simulink model "towing_project"  (Simulink 10.1)
settings: Solver=ode4  StartTime=0.0  StopTime=5000  FixedStep=1  RelTol=1e-3  EnableMultiTasking=on
PreLoadFcn:
  | load('Initialization_data.mat');
values from neighbouring files (symbols this model uses):
  D1 = [MM(1,1)/100, 0, 0; 0, MM(2,2)/40, 0; 0, 0, MM(3,3)/20]    [initail_data.m]
  M1 = diag([6.25e5, 6.25e5, 6.25e5*7.5^2])    [initail_data.m]    (also in msfunMotion_Display.m = makehgtform('translate',[block.Dwork(7).Data(1) block.Dwork()
  Ma1 = [7.58e4, 0, 0; 0, 3.69e5 -1.4e5; 0, -1.4e5, 8.77e6]    [initail_data.m]
  p00 = [0, 0, 0]'    [initail_data.m]
  p10 = [394, 237, 31]'    [initail_data.m]
  p20 = [394, -237, -31]'    [initail_data.m]
  p30 = [-394, -237, -149]'    [initail_data.m]
  p40 = [-394, 237, 149]'    [initail_data.m]
undefined symbols (not defined in the file or in its folder): D, M, Ma, magnitude
libraries: simulink x10, simulink_extras x4
(part 1 of 2)
settings Model: Creator=Lither  LastModifiedBy=Administrator
settings DataIOCC: LimitDataPoints=on
settings OptimizationCC: ExpressionDepthLimit=2147483647
settings DebuggingCC: FcnCallInpInsideContextMsg=warning  StateNameClashWarn=warning
settings ConfigComp: CovSFcnEnable=off

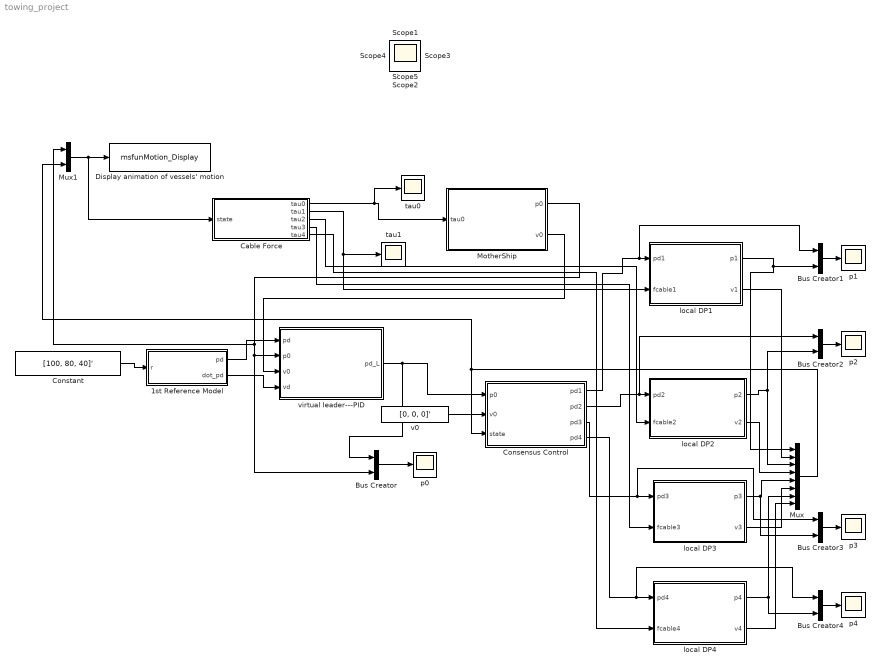
== system towing_project ==
  1st Reference Model : Subsystem  mask{T=200}
      mask prompts: T "Time constant of reference model"
  Bus Creator{,1..4} (5 alike) : BusCreator  Inputs=2
  Cable Force : MATLAB Function  TreatAsAtomicUnit=on
  Consensus Control : MATLAB Function  TreatAsAtomicUnit=on
  Constant : Constant  Value=[100, 80, 40]'
  Display animation of vessels' motion : M-S-Function  FunctionName=msfunMotion_Display  Parameters=p00, p10, p20, p30, p40
  MotherShip : Subsystem  mask{wv=on}
      mask prompts: wv "Display animation of the vessel's motion"
  Mux : Mux  Inputs=8
  Mux1 : Mux  Inputs=2
  local DP1 : Subsystem
  local DP2 : Subsystem
  local DP3 : Subsystem
  local DP4 : Subsystem
  p{0..4} (5 alike) : Scope
  tau0 : Scope
  tau1 : Scope
  v0 : Constant  Value=[0, 0, 0]'
  virtual leader---PID : Subsystem  mask{Kp_L=diag([0.8, 1, 0.8])*0.05, Kd_L=diag([1, 1, 1])*0.03, Ki_L=diag([1, 1, 1])*0.001}
      mask prompts: Kp_L "比例增益：Kp_L"; Kd_L "微分增益：Kd_L"; Ki_L "积分增益：Ki_L"
  Scope{,1..5} (6 alike) : Scope
  wires:
  Consensus Control/1(pd1) -> Bus Creator1/1, local DP1/1(pd1)
  local DP1/1(p1) -> Bus Creator1/2, Mux/1
  local DP1/2(v1) -> Mux/2
  local DP2/1(p2) -> Mux/3, Bus Creator2/2
  local DP2/2(v2) -> Mux/4
  Mux/1 -> Consensus Control/3(state), Mux1/2
  Consensus Control/2(pd2) -> Bus Creator2/1, local DP2/1(pd2)
  Mux1/1 -> Cable Force/1(state), Display animation of vessels' motion/1
  Constant/1 -> 1st Reference Model/1(r)
  local DP3/1(p3) -> Bus Creator3/2, Mux/5
  local DP3/2(v3) -> Mux/6
  local DP4/1(p4) -> Bus Creator4/2, Mux/7
  local DP4/2(v4) -> Mux/8
  Consensus Control/3(pd3) -> Bus Creator3/1, local DP3/1(pd3)
  Consensus Control/4(pd4) -> Bus Creator4/1, local DP4/1(pd4)
  1st Reference Model/1(pd) -> virtual leader---PID/1(pd)
  1st Reference Model/2(dot_pd) -> virtual leader---PID/4(vd)
  virtual leader---PID/1(pd_L) -> Bus Creator/1, Consensus Control/1(p0)
  v0/1 -> Consensus Control/2(v0)
  MotherShip/1(p0) -> Bus Creator/2, virtual leader---PID/2(p0), Mux1/1
  MotherShip/2(v0) -> virtual leader---PID/3(v0)
  Cable Force/1(tau0) -> tau0/1, MotherShip/1(tau0)
  Bus Creator/1 -> p0/1
  Cable Force/2(tau1) -> tau1/1, local DP1/2(fcable1)
  Cable Force/3(tau2) -> local DP2/2(fcable2)
  Cable Force/4(tau3) -> local DP3/2(fcable3)
  Cable Force/5(tau4) -> local DP4/2(fcable4)
  Bus Creator1/1 -> p1/1
  Bus Creator2/1 -> p2/1
  Bus Creator3/1 -> p3/1
  Bus Creator4/1 -> p4/1

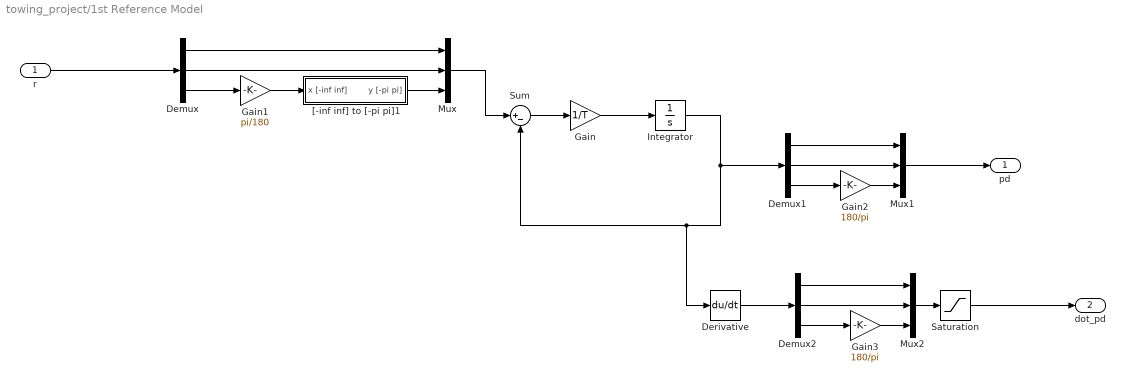
== system towing_project/1st Reference Model ==
  r : Inport
  Demux : Demux  Outputs=3
  Demux1 : Demux  Outputs=3
  Demux2 : Demux  Outputs=3
  Derivative : Derivative
  Gain : Gain  Gain=1/T
  Gain1 : Gain  Gain=pi/180
  Gain2 : Gain  Gain=180/pi
  Gain3 : Gain  Gain=180/pi
  Integrator : Integrator  InitialCondition=p00
  Mux : Mux  Inputs=3
  Mux1 : Mux  Inputs=3
  Mux2 : Mux  Inputs=3
  Saturation : Saturate  UpperLimit=10  LowerLimit=-10
  Sum : Sum  Inputs=|+-
  "[-inf inf] to [-pi pi]1" : Subsystem
  pd : Outport
  dot_pd : Outport  Port=2
  wires:
  Integrator/1 -> Derivative/1, Sum/2, Demux1/1
  Sum/1 -> Gain/1
  Gain/1 -> Integrator/1
  Saturation/1 -> dot_pd/1
  r/1 -> Demux/1
  Demux/3 -> Gain1/1
  Demux/2 -> Mux/2
  Demux/1 -> Mux/1
  Mux/1 -> Sum/1
  Demux1/3 -> Gain2/1
  Gain2/1 -> Mux1/3
  Demux1/2 -> Mux1/2
  Demux1/1 -> Mux1/1
  Mux1/1 -> pd/1
  Demux2/3 -> Gain3/1
  Demux2/2 -> Mux2/2
  Demux2/1 -> Mux2/1
  Gain3/1 -> Mux2/3
  Derivative/1 -> Demux2/1
  Mux2/1 -> Saturation/1
  Gain1/1 -> "[-inf inf] to [-pi pi]1"/1(x [-inf inf])
  "[-inf inf] to [-pi pi]1"/1(y [-pi pi]) -> Mux/3

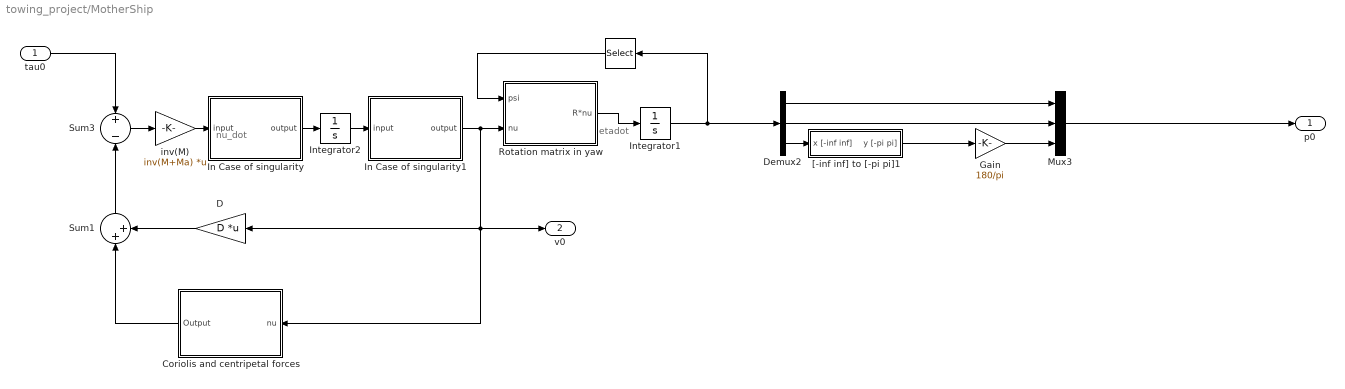
== system towing_project/MotherShip ==
  note: nu_dot
  note: etadot
  tau0 : Inport
  " " : Selector  InputPortWidth=3  IndexOptions=Index vector (dialog)  Indices=[3]  OutputSizes=1
  Coriolis and centripetal forces : Subsystem
  D : Gain  Gain=D  Multiplication=Matrix(K*u)  SaturateOnIntegerOverflow=on  OutDataTypeStr=Inherit: Same as input  ParamDataTypeStr=Inherit: Same as input
  Demux2 : Demux  Outputs=3
  Gain : Gain  Gain=180/pi
  In Case of singularity : Subsystem
  In Case of singularity1 : Subsystem
  Integrator1 : Integrator  InitialCondition=[p00(1), p00(2), p00(3)/180*pi]'
  Integrator2 : Integrator
  Mux3 : Mux  Inputs=3
  Rotation matrix in yaw : Subsystem
  Sum1 : Sum  Inputs=|++  InputSameDT=on  SaturateOnIntegerOverflow=on  OutDataTypeStr=Inherit: Same as first input
  Sum3 : Sum  Inputs=+-  InputSameDT=on  SaturateOnIntegerOverflow=on  OutDataTypeStr=Inherit: Same as first input
  "[-inf inf] to [-pi pi]1" : Subsystem
  inv(M) : Gain  Gain=inv(M+Ma)  Multiplication=Matrix(K*u)  SaturateOnIntegerOverflow=on  OutDataTypeStr=Inherit: Same as input  ParamDataTypeStr=Inherit: Same as input
  p0 : Outport
  v0 : Outport  Port=2
  wires:
  Sum3/1 -> inv(M)/1
  inv(M)/1 -> In Case of singularity/1(input)
  Rotation matrix in yaw/1(R*nu) -> Integrator1/1
  Integrator1/1 -> Demux2/1, " "/1
  " "/1 -> Rotation matrix in yaw/1(psi)
  tau0/1 -> Sum3/1
  Integrator2/1 -> In Case of singularity1/1(input)
  In Case of singularity/1(output) -> Integrator2/1
  In Case of singularity1/1(output) -> Rotation matrix in yaw/2(nu), D/1, Coriolis and centripetal forces/1(nu), v0/1
  D/1 -> Sum1/2
  Coriolis and centripetal forces/1(Output) -> Sum1/1
  Sum1/1 -> Sum3/2
  Demux2/3 -> "[-inf inf] to [-pi pi]1"/1(x [-inf inf])
  Demux2/1 -> Mux3/1
  Demux2/2 -> Mux3/2
  Mux3/1 -> p0/1
  "[-inf inf] to [-pi pi]1"/1(y [-pi pi]) -> Gain/1
  Gain/1 -> Mux3/3

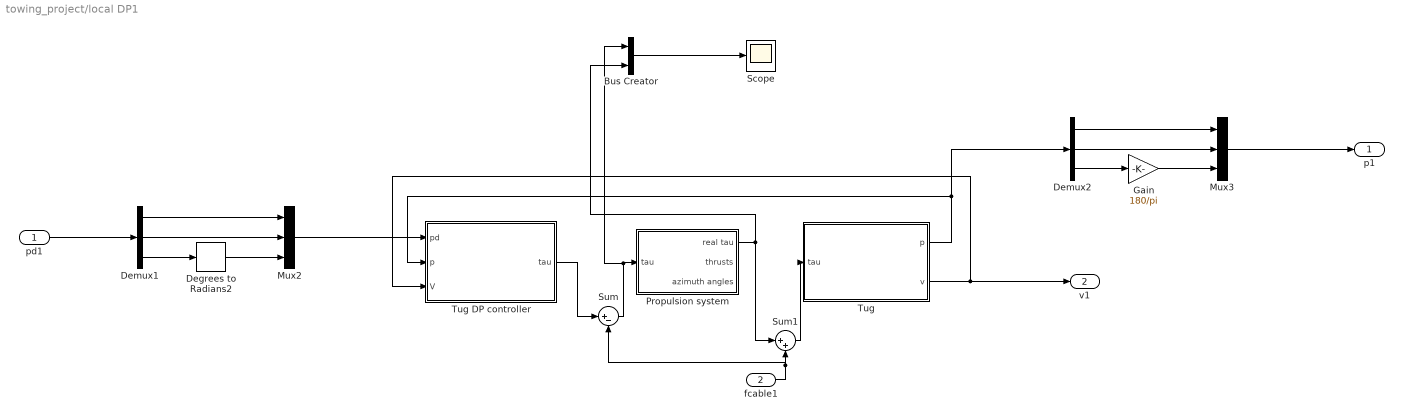
== system towing_project/local DP1 ==
  pd1 : Inport
  fcable1 : Inport  Port=2
  Bus Creator : BusCreator  Inputs=2
  Degrees to Radians2 : simulink_extras/Transformations/Degrees to Radians
  Demux1 : Demux  Outputs=3
  Demux2 : Demux  Outputs=3
  Gain : Gain  Gain=180/pi
  Mux2 : Mux  Inputs=3
  Mux3 : Mux  Inputs=3
  Propulsion system : Subsystem  mask{f0=[1;1;1], a0=[5;6;7], u0=[1; 1; 1], wa=on}
      mask prompts: f0 "Initial values of thrusts"; a0 "Initial values of azimuth angles"; u0 "Thruster utilization"; wa "Show animation of thrust and azimuth angle"
  Scope : Scope
  Sum : Sum  Inputs=|+-
  Sum1 : Sum  Inputs=|++
  Tug : Subsystem  mask{wv=on}
      mask prompts: wv "Display animation of the vessel's motion"
  Tug DP controller : Subsystem  mask(Nonlinear DP Controller){Kp=diag([0.0028, 0.004, 0.0031]), Kd=diag([0.0573, 0.0716, 0.025]), Ki=diag([0.0028, 0.004, 0.0031])*0.01, WFF_gain=0}
      mask prompts: Kp "Proportional Gain Matrix: Kp"; Kd "Derivative Gain Matrix: Kd"; Ki "Integral Gain Matrix: Ki"; WFF_gain "Wave feedforward Gain"
      mask help: PID controller for Set-Point Reulation in Surge, Sway and Yaw
      mask Help:
      | The nonlinear  PID controller uses the rotation matrix in yaw for proper scaling of the surge, sway and yaw gains as a function of the yaw angle.
      | INPUTS: (1) eta_ref, (2) eta, (3) nu. OUPUTS: (1) tau.
      mask Display: disp('PID controller')
  p1 : Outport
  v1 : Outport  Port=2
  wires:
  Tug/2(v) -> v1/1, Tug DP controller/3(V)
  Demux1/2 -> Mux2/2
  Mux2/1 -> Tug DP controller/1(pd)
  Demux1/1 -> Mux2/1
  Degrees to Radians2/1 -> Mux2/3
  Demux1/3 -> Degrees to Radians2/1
  pd1/1 -> Demux1/1
  Demux2/2 -> Mux3/2
  Tug/1(p) -> Demux2/1, Tug DP controller/2(p)
  Mux3/1 -> p1/1
  Demux2/3 -> Gain/1
  Gain/1 -> Mux3/3
  Demux2/1 -> Mux3/1
  Tug DP controller/1(tau) -> Sum/1
  Sum/1 -> Bus Creator/1, Propulsion system/1(tau)
  fcable1/1 -> Sum/2, Sum1/2
  Propulsion system/1(real tau) -> Sum1/1, Bus Creator/2
  Sum1/1 -> Tug/1(tau)
  Bus Creator/1 -> Scope/1

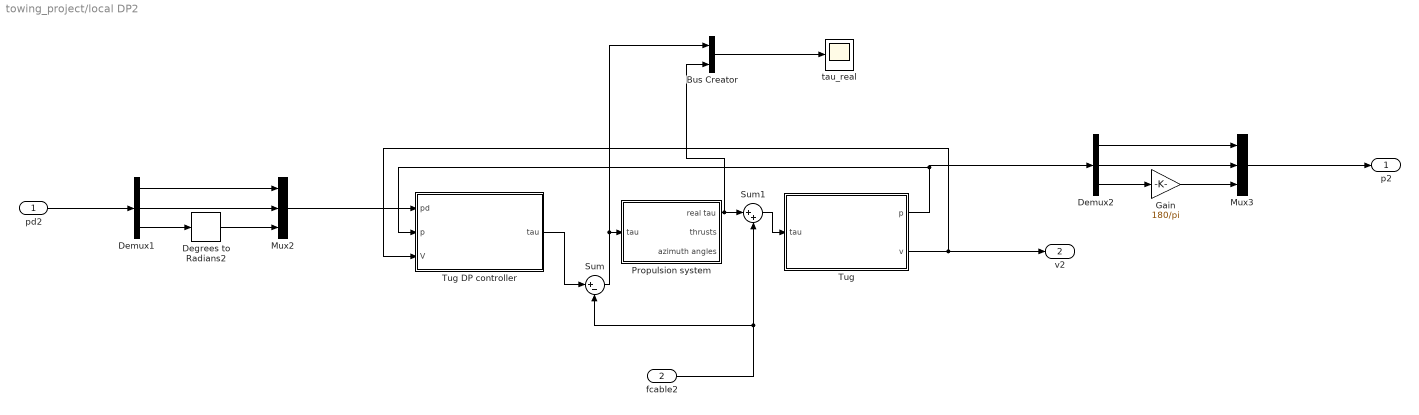
== system towing_project/local DP2 ==
  pd2 : Inport
  fcable2 : Inport  Port=2
  Bus Creator : BusCreator  Inputs=2
  Degrees to Radians2 : simulink_extras/Transformations/Degrees to Radians
  Demux1 : Demux  Outputs=3
  Demux2 : Demux  Outputs=3
  Gain : Gain  Gain=180/pi
  Mux2 : Mux  Inputs=3
  Mux3 : Mux  Inputs=3
  Propulsion system : Subsystem  mask{f0=[1;1;1], a0=[50;60;70], u0=[1; 1; 1], wa=on}
      mask prompts: f0 "Initial values of thrusts"; a0 "Initial values of azimuth angles"; u0 "Thruster utilization"; wa "Show animation of thrust and azimuth angle"
  Sum : Sum  Inputs=|+-
  Sum1 : Sum  Inputs=|++
  Tug : Subsystem  mask{wv=on}
      mask prompts: wv "Display animation of the vessel's motion"
  Tug DP controller : Subsystem  mask(Nonlinear DP Controller){Kp=diag([0.0028, 0.004, 0.0031]), Kd=diag([0.0573, 0.0716, 0.025]), Ki=diag([0.0028, 0.004, 0.0031])*0.01, WFF_gain=0}
      mask prompts: Kp "Proportional Gain Matrix: Kp"; Kd "Derivative Gain Matrix: Kd"; Ki "Integral Gain Matrix: Ki"; WFF_gain "Wave feedforward Gain"
      mask help: PID controller for Set-Point Reulation in Surge, Sway and Yaw
      mask Help:
      | The nonlinear  PID controller uses the rotation matrix in yaw for proper scaling of the surge, sway and yaw gains as a function of the yaw angle.
      | INPUTS: (1) eta_ref, (2) eta, (3) nu. OUPUTS: (1) tau.
      mask Display: disp('PID controller')
  tau_real : Scope
  p2 : Outport
  v2 : Outport  Port=2
  wires:
  Tug/2(v) -> v2/1, Tug DP controller/3(V)
  Demux1/2 -> Mux2/2
  Mux2/1 -> Tug DP controller/1(pd)
  Demux1/1 -> Mux2/1
  Degrees to Radians2/1 -> Mux2/3
  Demux1/3 -> Degrees to Radians2/1
  pd2/1 -> Demux1/1
  Mux3/1 -> p2/1
  Tug/1(p) -> Demux2/1, Tug DP controller/2(p)
  Demux2/3 -> Gain/1
  Demux2/2 -> Mux3/2
  Gain/1 -> Mux3/3
  Demux2/1 -> Mux3/1
  Propulsion system/1(real tau) -> Bus Creator/2, Sum1/1
  Sum1/1 -> Tug/1(tau)
  fcable2/1 -> Sum/2, Sum1/2
  Tug DP controller/1(tau) -> Sum/1
  Sum/1 -> Bus Creator/1, Propulsion system/1(tau)
  Bus Creator/1 -> tau_real/1

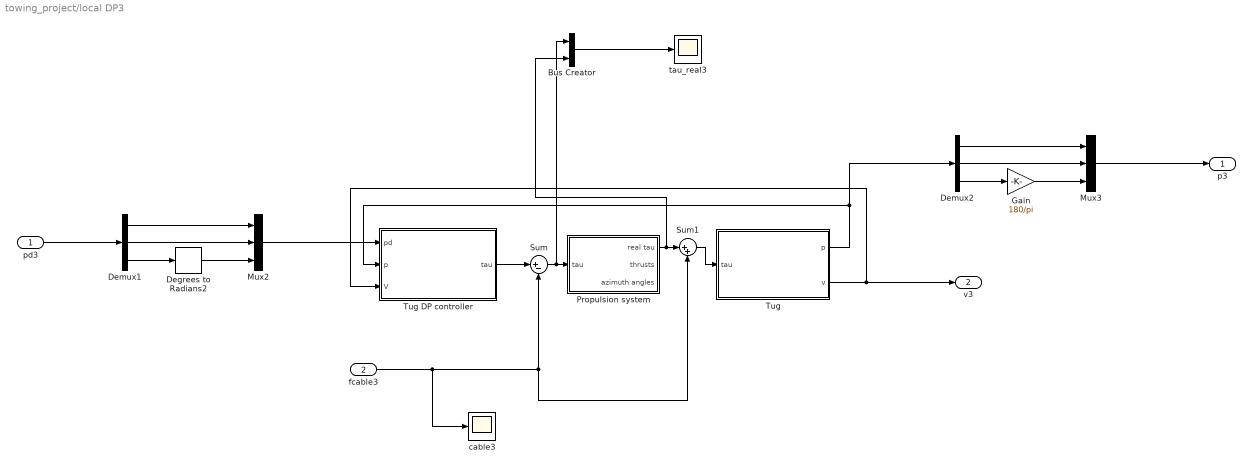
== system towing_project/local DP3 ==
  pd3 : Inport
  fcable3 : Inport  Port=2
  Bus Creator : BusCreator  Inputs=2
  Degrees to Radians2 : simulink_extras/Transformations/Degrees to Radians
  Demux1 : Demux  Outputs=3
  Demux2 : Demux  Outputs=3
  Gain : Gain  Gain=180/pi
  Mux2 : Mux  Inputs=3
  Mux3 : Mux  Inputs=3
  Propulsion system : Subsystem  mask{f0=[1;1;1], a0=[50;60;70], u0=[1; 1; 1], wa=on}
      mask prompts: f0 "Initial values of thrusts"; a0 "Initial values of azimuth angles"; u0 "Thruster utilization"; wa "Show animation of thrust and azimuth angle"
  Sum : Sum  Inputs=|+-
  Sum1 : Sum  Inputs=|++
  Tug : Subsystem  mask{wv=on}
      mask prompts: wv "Display animation of the vessel's motion"
  Tug DP controller : Subsystem  mask(Nonlinear DP Controller){Kp=diag([0.0028, 0.004, 0.0031]), Kd=diag([0.0573, 0.0716, 0.025]), Ki=diag([0.0028, 0.004, 0.0031])*0.01, WFF_gain=0}
      mask prompts: Kp "Proportional Gain Matrix: Kp"; Kd "Derivative Gain Matrix: Kd"; Ki "Integral Gain Matrix: Ki"; WFF_gain "Wave feedforward Gain"
      mask help: PID controller for Set-Point Reulation in Surge, Sway and Yaw
      mask Help:
      | The nonlinear  PID controller uses the rotation matrix in yaw for proper scaling of the surge, sway and yaw gains as a function of the yaw angle.
      | INPUTS: (1) eta_ref, (2) eta, (3) nu. OUPUTS: (1) tau.
      mask Display: disp('PID controller')
  cable3 : Scope
  tau_real3 : Scope
  p3 : Outport
  v3 : Outport  Port=2
  wires:
  Tug/2(v) -> v3/1, Tug DP controller/3(V)
  Demux1/2 -> Mux2/2
  Mux2/1 -> Tug DP controller/1(pd)
  Demux1/1 -> Mux2/1
  Degrees to Radians2/1 -> Mux2/3
  Demux1/3 -> Degrees to Radians2/1
  pd3/1 -> Demux1/1
  Demux2/2 -> Mux3/2
  Tug/1(p) -> Demux2/1, Tug DP controller/2(p)
  Mux3/1 -> p3/1
  Demux2/3 -> Gain/1
  Gain/1 -> Mux3/3
  Demux2/1 -> Mux3/1
  Propulsion system/1(real tau) -> Bus Creator/2, Sum1/1
  Sum1/1 -> Tug/1(tau)
  fcable3/1 -> cable3/1, Sum1/2, Sum/2
  Tug DP controller/1(tau) -> Sum/1
  Sum/1 -> Bus Creator/1, Propulsion system/1(tau)
  Bus Creator/1 -> tau_real3/1

== system towing_project/local DP4 ==
  pd4 : Inport
  fcable4 : Inport  Port=2
  Degrees to Radians2 : simulink_extras/Transformations/Degrees to Radians
  Demux1 : Demux  Outputs=3
  Demux2 : Demux  Outputs=3
  Gain : Gain  Gain=180/pi
  Mux2 : Mux  Inputs=3
  Mux3 : Mux  Inputs=3
  Propulsion system : Subsystem  mask{f0=[1;1;1], a0=[50;60;70], u0=[1; 1; 1], wa=on}
      mask prompts: f0 "Initial values of thrusts"; a0 "Initial values of azimuth angles"; u0 "Thruster utilization"; wa "Show animation of thrust and azimuth angle"
  Sum : Sum  Inputs=|+-
  Sum1 : Sum  Inputs=|++
  Tug : Subsystem  mask{wv=on}
      mask prompts: wv "Display animation of the vessel's motion"
  Tug DP controller : Subsystem  mask(Nonlinear DP Controller){Kp=diag([0.0028, 0.004, 0.0031]), Kd=diag([0.0573, 0.0716, 0.025]), Ki=diag([0.0028, 0.004, 0.0031])*0.01, WFF_gain=0}
      mask prompts: Kp "Proportional Gain Matrix: Kp"; Kd "Derivative Gain Matrix: Kd"; Ki "Integral Gain Matrix: Ki"; WFF_gain "Wave feedforward Gain"
      mask help: PID controller for Set-Point Reulation in Surge, Sway and Yaw
      mask Help:
      | The nonlinear  PID controller uses the rotation matrix in yaw for proper scaling of the surge, sway and yaw gains as a function of the yaw angle.
      | INPUTS: (1) eta_ref, (2) eta, (3) nu. OUPUTS: (1) tau.
      mask Display: disp('PID controller')
  p4 : Outport
  v4 : Outport  Port=2
  wires:
  Tug/2(v) -> v4/1, Tug DP controller/3(V)
  Demux1/2 -> Mux2/2
  Mux2/1 -> Tug DP controller/1(pd)
  Demux1/1 -> Mux2/1
  Degrees to Radians2/1 -> Mux2/3
  Demux1/3 -> Degrees to Radians2/1
  pd4/1 -> Demux1/1
  Demux2/2 -> Mux3/2
  Tug/1(p) -> Demux2/1, Tug DP controller/2(p)
  Mux3/1 -> p4/1
  Demux2/3 -> Gain/1
  Gain/1 -> Mux3/3
  Demux2/1 -> Mux3/1
  Propulsion system/1(real tau) -> Sum1/1
  Sum1/1 -> Tug/1(tau)
  fcable4/1 -> Sum/2, Sum1/2
  Tug DP controller/1(tau) -> Sum/1
  Sum/1 -> Propulsion system/1(tau)

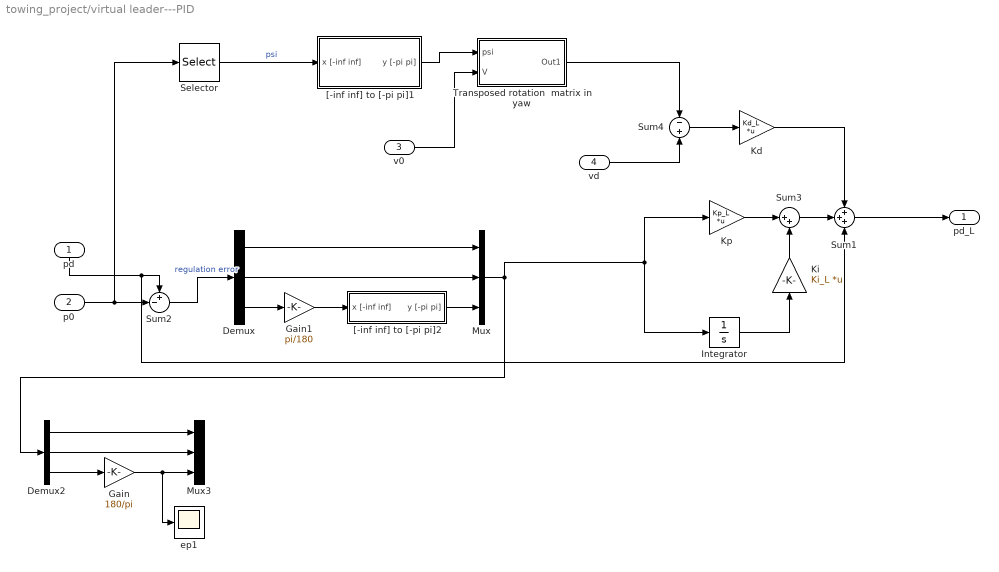
== system towing_project/virtual leader---PID ==
  pd : Inport
  p0 : Inport  Port=2
  v0 : Inport  Port=3
  vd : Inport  Port=4
  Demux : Demux  Outputs=3
  Demux2 : Demux  Outputs=3
  Gain : Gain  Gain=180/pi
  Gain1 : Gain  Gain=pi/180
  Integrator : Integrator
  Kd : Gain  Gain=Kd_L  Multiplication=Matrix(K*u)  SaturateOnIntegerOverflow=on  OutDataTypeStr=Inherit: Same as input  ParamDataTypeStr=Inherit: Same as input
  Ki : Gain  Gain=Ki_L  Multiplication=Matrix(K*u)  SaturateOnIntegerOverflow=on  OutDataTypeStr=Inherit: Same as input  ParamDataTypeStr=Inherit: Same as input
  Kp : Gain  Gain=Kp_L  Multiplication=Matrix(K*u)  SaturateOnIntegerOverflow=on  OutDataTypeStr=Inherit: Same as input  ParamDataTypeStr=Inherit: Same as input
  Mux : Mux  Inputs=3
  Mux3 : Mux  Inputs=3
  Selector : Selector  InputPortWidth=3  IndexOptions=Index vector (dialog)  Indices=[ 3]  OutputSizes=1
  Sum1 : Sum  Inputs=+++  InputSameDT=on  SaturateOnIntegerOverflow=on  OutDataTypeStr=Inherit: Same as first input
  Sum2 : Sum  Inputs=+-|  InputSameDT=on  SaturateOnIntegerOverflow=on  OutDataTypeStr=Inherit: Same as first input
  Sum3 : Sum  Inputs=|++  InputSameDT=on  SaturateOnIntegerOverflow=on  OutDataTypeStr=Inherit: Same as first input
  Sum4 : Sum  Inputs=-+  InputSameDT=on  SaturateOnIntegerOverflow=on  OutDataTypeStr=Inherit: Same as first input
  Transposed rotation  matrix in yaw : Subsystem
  "[-inf inf] to [-pi pi]1" : Subsystem
  "[-inf inf] to [-pi pi]2" : Subsystem
  ep1 : Scope
  pd_L : Outport  InitialOutput=0
  wires:
  Gain/1 -> ep1/1, Mux3/3
  Demux2/1 -> Mux3/1
  Kp/1 -> Sum3/1
  "[-inf inf] to [-pi pi]1"/1(y [-pi pi]) -> Transposed rotation  matrix in yaw/1(psi)
  Demux2/3 -> Gain/1
  Demux2/2 -> Mux3/2
  Integrator/1 -> Ki/1
  Sum1/1 -> pd_L/1
  p0/1 -> Sum2/2, Selector/1
  Sum2/1 -> Demux/1  "regulation error"
  pd/1 -> Sum1/3, Sum2/1
  Mux/1 -> Demux2/1, Kp/1, Integrator/1
  Demux/1 -> Mux/1
  Selector/1 -> "[-inf inf] to [-pi pi]1"/1(x [-inf inf])  "psi"
  Ki/1 -> Sum3/2
  Demux/2 -> Mux/2
  "[-inf inf] to [-pi pi]2"/1(y [-pi pi]) -> Mux/3
  Demux/3 -> Gain1/1
  Gain1/1 -> "[-inf inf] to [-pi pi]2"/1(x [-inf inf])
  v0/1 -> Transposed rotation  matrix in yaw/2(V)
  Sum4/1 -> Kd/1
  Kd/1 -> Sum1/1
  Sum3/1 -> Sum1/2
  Transposed rotation  matrix in yaw/1(Out1) -> Sum4/1
  vd/1 -> Sum4/2

== system towing_project/1st Reference Model/[-inf inf] to [-pi pi]1 ==
  note: x
  note: r
  x [-inf inf] : Inport
  Constant : Constant  Value=2*pi
  Gain : Gain  Gain=pi  SaturateOnIntegerOverflow=on  OutDataTypeStr=Inherit: Same as input  ParamDataTypeStr=Inherit: Same as input
  Math Function : Math  Operator=rem  SignedPower=on  SaturateOnIntegerOverflow=on
  Saturation : Saturate  UpperLimit=1e10  LowerLimit=-1e10
  Sign : Signum
  Sum : Sum  Inputs=|+-  SaturateOnIntegerOverflow=on
  Sum1 : Sum  Inputs=|++  SaturateOnIntegerOverflow=on
  y [-pi pi] : Outport
  wires:
  x [-inf inf]/1 -> Saturation/1
  Sign/1 -> Gain/1
  Gain/1 -> Sum/2, Sum1/2
  Sum1/1 -> Math Function/1
  Constant/1 -> Math Function/2
  Math Function/1 -> Sum/1
  Sum/1 -> y [-pi pi]/1
  Saturation/1 -> Sum1/1, Sign/1

== system towing_project/MotherShip/Coriolis and centripetal forces ==
  nu : Inport
  Mux : Mux  Inputs=3
  Selector1 : Selector  InputPortWidth=3  IndexOptions=Index vector (dialog)  Indices=[1 ]  OutputSizes=1
  Selector2 : Selector  InputPortWidth=3  IndexOptions=Index vector (dialog)  Indices=[2]  OutputSizes=1
  Selector3 : Selector  InputPortWidth=3  IndexOptions=Index vector (dialog)  Indices=[3]  OutputSizes=1
  Subsystem : Subsystem
  Subsystem1 : Subsystem
  Subsystem2 : Subsystem
  Output : Outport
  wires:
  nu/1 -> Selector1/1, Selector2/1, Selector3/1
  Selector2/1 -> Subsystem/1(v), Subsystem2/2(v)  "v"
  Selector3/1 -> Subsystem/2(r), Subsystem1/2(r), Subsystem2/3(r)  "r"
  Selector1/1 -> Subsystem1/1(u), Subsystem2/1(u)  "u"
  Subsystem/1(x direction) -> Mux/1
  Subsystem1/1(y direction) -> Mux/2
  Subsystem2/1(yaw direction) -> Mux/3
  Mux/1 -> Output/1

== system towing_project/MotherShip/In Case of singularity ==
  input : Inport
  Compare To Constant : simulink/Logic and Bit Operations/Compare To Constant  relop=>=  const=1e8  OutDataTypeStr=boolean
  Stop Simulation : Stop
  output : Outport
  wires:
  input/1 -> output/1, Compare To Constant/1
  Compare To Constant/1 -> Stop Simulation/1

== system towing_project/MotherShip/In Case of singularity1 ==
  input : Inport
  Compare To Constant : simulink/Logic and Bit Operations/Compare To Constant  relop=>=  const=1e10  OutDataTypeStr=boolean
  Stop Simulation : Stop
  output : Outport
  wires:
  input/1 -> output/1, Compare To Constant/1
  Compare To Constant/1 -> Stop Simulation/1

== system towing_project/MotherShip/Rotation matrix in yaw ==
  psi : Inport
  nu : Inport  Port=2
  Fcn : Fcn  Expr=cos(u(1))*u(2)-sin(u(1))*u(3)
  Fcn1 : Fcn  Expr=sin(u(1))*u(2)+cos(u(1))*u(3)
  Fcn2 : Fcn  Expr=u(4)
  Mux : Mux  Inputs=2
  Mux1 : Mux  Inputs=3
  R*nu : Outport
  wires:
  Mux1/1 -> R*nu/1  "eta_dot"
  Mux/1 -> Fcn/1, Fcn1/1, Fcn2/1
  psi/1 -> Mux/1
  nu/1 -> Mux/2
  Fcn1/1 -> Mux1/2  "y_dot"
  Fcn/1 -> Mux1/1  "x_dot"
  Fcn2/1 -> Mux1/3  "psi_dot"

== system towing_project/MotherShip/[-inf inf] to [-pi pi]1 ==
  note: x
  note: r
  x [-inf inf] : Inport
  Constant : Constant  Value=2*pi
  Gain : Gain  Gain=pi  SaturateOnIntegerOverflow=on  OutDataTypeStr=Inherit: Same as input  ParamDataTypeStr=Inherit: Same as input
  Math Function : Math  Operator=rem  SignedPower=on  SaturateOnIntegerOverflow=on
  Saturation : Saturate  UpperLimit=1e10  LowerLimit=-1e10
  Sign : Signum
  Sum : Sum  Inputs=|+-  SaturateOnIntegerOverflow=on
  Sum1 : Sum  Inputs=|++  SaturateOnIntegerOverflow=on
  y [-pi pi] : Outport
  wires:
  x [-inf inf]/1 -> Saturation/1
  Sign/1 -> Gain/1
  Gain/1 -> Sum/2, Sum1/2
  Sum1/1 -> Math Function/1
  Constant/1 -> Math Function/2
  Math Function/1 -> Sum/1
  Sum/1 -> y [-pi pi]/1
  Saturation/1 -> Sum1/1, Sign/1

== system towing_project/local DP1/Propulsion system ==
  tau : Inport
  AzimuthAngle1 : ToWorkspace  VariableName=AziAng1  SampleTime=-1
  Gain : Gain  Gain=1/1000
  Gain1 : Gain  Gain=1000
  Level-2 MATLAB S-Function : M-S-Function  FunctionName=msfunTA_PA  Parameters=f0,a0,wa
  RealTau : ToWorkspace  VariableName=RealTau1  SampleTime=-1
  Terminator : Terminator
  Terminator1 : Terminator
  Terminator2 : Terminator
  ThrusterForce : ToWorkspace  VariableName=Thrust1  SampleTime=-1
  real tau : Outport
  thrusts : Outport  Port=2
  azimuth angles : Outport  Port=3
  wires:
  tau/1 -> Gain/1
  Level-2 MATLAB S-Function/2 -> Terminator/1
  Level-2 MATLAB S-Function/3 -> AzimuthAngle1/1, azimuth angles/1
  Level-2 MATLAB S-Function/4 -> Terminator1/1
  Level-2 MATLAB S-Function/5 -> Gain1/1
  Level-2 MATLAB S-Function/6 -> Terminator2/1
  Level-2 MATLAB S-Function/1 -> ThrusterForce/1, thrusts/1
  Gain/1 -> Level-2 MATLAB S-Function/1
  Gain1/1 -> RealTau/1, real tau/1

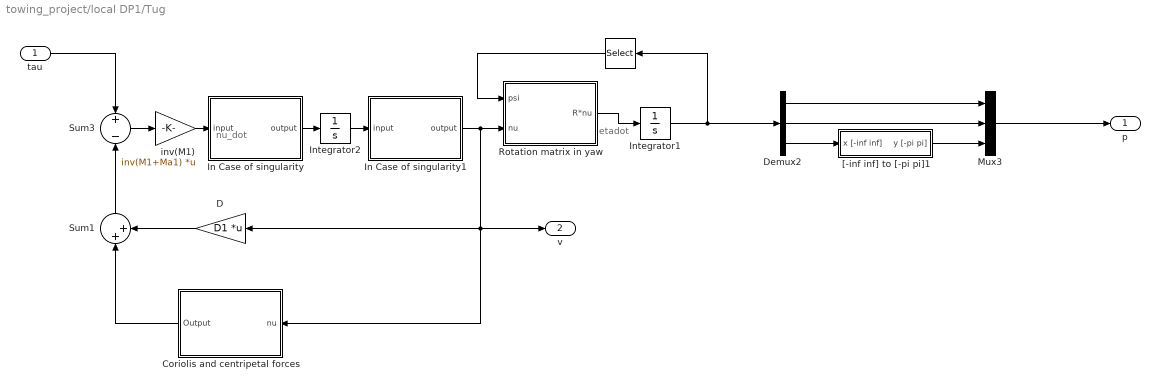
== system towing_project/local DP1/Tug ==
  note: nu_dot
  note: etadot
  tau : Inport
  " " : Selector  InputPortWidth=3  IndexOptions=Index vector (dialog)  Indices=[3]  OutputSizes=1
  Coriolis and centripetal forces : Subsystem
  D : Gain  Gain=D1  Multiplication=Matrix(K*u)  SaturateOnIntegerOverflow=on  OutDataTypeStr=Inherit: Same as input  ParamDataTypeStr=Inherit: Same as input
  Demux2 : Demux  Outputs=3
  In Case of singularity : Subsystem
  In Case of singularity1 : Subsystem
  Integrator1 : Integrator  InitialCondition=[p10(1), p10(2), p10(3)/180*pi]'
  Integrator2 : Integrator
  Mux3 : Mux  Inputs=3
  Rotation matrix in yaw : Subsystem
  Sum1 : Sum  Inputs=|++  InputSameDT=on  SaturateOnIntegerOverflow=on  OutDataTypeStr=Inherit: Same as first input
  Sum3 : Sum  Inputs=+-  InputSameDT=on  SaturateOnIntegerOverflow=on  OutDataTypeStr=Inherit: Same as first input
  "[-inf inf] to [-pi pi]1" : Subsystem
  inv(M1) : Gain  Gain=inv(M1+Ma1)  Multiplication=Matrix(K*u)  SaturateOnIntegerOverflow=on  OutDataTypeStr=Inherit: Same as input  ParamDataTypeStr=Inherit: Same as input
  p : Outport
  v : Outport  Port=2
  wires:
  Sum3/1 -> inv(M1)/1
  inv(M1)/1 -> In Case of singularity/1(input)
  Rotation matrix in yaw/1(R*nu) -> Integrator1/1
  Integrator1/1 -> Demux2/1, " "/1
  " "/1 -> Rotation matrix in yaw/1(psi)
  tau/1 -> Sum3/1
  Integrator2/1 -> In Case of singularity1/1(input)
  In Case of singularity/1(output) -> Integrator2/1
  In Case of singularity1/1(output) -> Rotation matrix in yaw/2(nu), D/1, Coriolis and centripetal forces/1(nu), v/1
  D/1 -> Sum1/2
  Coriolis and centripetal forces/1(Output) -> Sum1/1
  Sum1/1 -> Sum3/2
  Demux2/3 -> "[-inf inf] to [-pi pi]1"/1(x [-inf inf])
  Demux2/1 -> Mux3/1
  Demux2/2 -> Mux3/2
  "[-inf inf] to [-pi pi]1"/1(y [-pi pi]) -> Mux3/3
  Mux3/1 -> p/1

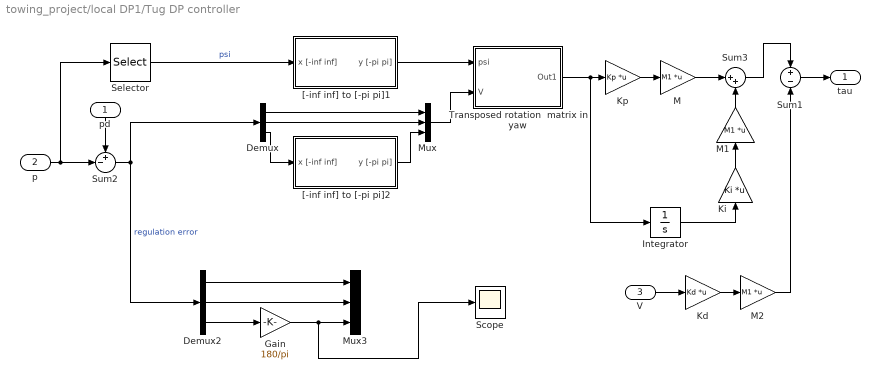
== system towing_project/local DP1/Tug DP controller ==
  pd : Inport
  p : Inport  Port=2
  V : Inport  Port=3
  Demux : Demux  Outputs=3
  Demux2 : Demux  Outputs=3
  Gain : Gain  Gain=180/pi
  Integrator : Integrator
  Kd : Gain  Gain=Kd  Multiplication=Matrix(K*u)  SaturateOnIntegerOverflow=on  OutDataTypeStr=Inherit: Same as input  ParamDataTypeStr=Inherit: Same as input
  Ki : Gain  Gain=Ki  Multiplication=Matrix(K*u)  SaturateOnIntegerOverflow=on  OutDataTypeStr=Inherit: Same as input  ParamDataTypeStr=Inherit: Same as input
  Kp : Gain  Gain=Kp  Multiplication=Matrix(K*u)  SaturateOnIntegerOverflow=on  OutDataTypeStr=Inherit: Same as input  ParamDataTypeStr=Inherit: Same as input
  M : Gain  Gain=M1  Multiplication=Matrix(K*u)  SaturateOnIntegerOverflow=on  OutDataTypeStr=Inherit: Same as input  ParamDataTypeStr=Inherit: Same as input
  M1 : Gain  Gain=M1  Multiplication=Matrix(K*u)  SaturateOnIntegerOverflow=on  OutDataTypeStr=Inherit: Same as input  ParamDataTypeStr=Inherit: Same as input
  M2 : Gain  Gain=M1  Multiplication=Matrix(K*u)  SaturateOnIntegerOverflow=on  OutDataTypeStr=Inherit: Same as input  ParamDataTypeStr=Inherit: Same as input
  Mux : Mux  Inputs=3
  Mux3 : Mux  Inputs=3
  Scope : Scope
  Selector : Selector  InputPortWidth=3  IndexOptions=Index vector (dialog)  Indices=[ 3]  OutputSizes=1
  Sum1 : Sum  Inputs=+-  InputSameDT=on  SaturateOnIntegerOverflow=on  OutDataTypeStr=Inherit: Same as first input
  Sum2 : Sum  Inputs=+-|  InputSameDT=on  SaturateOnIntegerOverflow=on  OutDataTypeStr=Inherit: Same as first input
  Sum3 : Sum  Inputs=|++  InputSameDT=on  SaturateOnIntegerOverflow=on  OutDataTypeStr=Inherit: Same as first input
  Transposed rotation  matrix in yaw : Subsystem
  "[-inf inf] to [-pi pi]1" : Subsystem
  "[-inf inf] to [-pi pi]2" : Subsystem
  tau : Outport  InitialOutput=0
  wires:
  "[-inf inf] to [-pi pi]1"/1(y [-pi pi]) -> Transposed rotation  matrix in yaw/1(psi)
  Selector/1 -> "[-inf inf] to [-pi pi]1"/1(x [-inf inf])  "psi"
  Mux/1 -> Transposed rotation  matrix in yaw/2(V)
  Demux/1 -> Mux/1
  Demux/2 -> Mux/2
  "[-inf inf] to [-pi pi]2"/1(y [-pi pi]) -> Mux/3
  Sum2/1 -> Demux2/1, Demux/1  "regulation error"
  Demux/3 -> "[-inf inf] to [-pi pi]2"/1(x [-inf inf])
  pd/1 -> Sum2/1
  Sum1/1 -> tau/1
  p/1 -> Sum2/2, Selector/1
  V/1 -> Kd/1
  Integrator/1 -> Ki/1
  Kp/1 -> M/1
  Ki/1 -> M1/1
  Transposed rotation  matrix in yaw/1(Out1) -> Kp/1, Integrator/1
  Kd/1 -> M2/1
  M/1 -> Sum3/1
  M1/1 -> Sum3/2
  Sum3/1 -> Sum1/1
  M2/1 -> Sum1/2
  Demux2/3 -> Gain/1
  Demux2/1 -> Mux3/1
  Demux2/2 -> Mux3/2
  Gain/1 -> Scope/1, Mux3/3

== system towing_project/local DP2/Propulsion system ==
  tau : Inport
  AzimuthAngle2 : ToWorkspace  VariableName=AziAng2  SampleTime=-1
  Gain : Gain  Gain=1/1000
  Gain1 : Gain  Gain=1000
  Level-2 MATLAB S-Function : M-S-Function  FunctionName=msfunTA_PA  Parameters=f0,a0,wa
  RealTau : ToWorkspace  VariableName=RealTau2  SampleTime=-1
  Terminator : Terminator
  Terminator1 : Terminator
  Terminator2 : Terminator
  ThrusterForce : ToWorkspace  VariableName=Thrust2  SampleTime=-1
  real tau : Outport
  thrusts : Outport  Port=2
  azimuth angles : Outport  Port=3
  wires:
  tau/1 -> Gain/1
  Level-2 MATLAB S-Function/2 -> Terminator/1
  Level-2 MATLAB S-Function/3 -> AzimuthAngle2/1, azimuth angles/1
  Level-2 MATLAB S-Function/4 -> Terminator1/1
  Level-2 MATLAB S-Function/5 -> Gain1/1
  Level-2 MATLAB S-Function/6 -> Terminator2/1
  Level-2 MATLAB S-Function/1 -> ThrusterForce/1, thrusts/1
  Gain/1 -> Level-2 MATLAB S-Function/1
  Gain1/1 -> RealTau/1, real tau/1

== system towing_project/local DP2/Tug ==
  note: nu_dot
  note: etadot
  tau : Inport
  " " : Selector  InputPortWidth=3  IndexOptions=Index vector (dialog)  Indices=[3]  OutputSizes=1
  Coriolis and centripetal forces : Subsystem
  D : Gain  Gain=D1  Multiplication=Matrix(K*u)  SaturateOnIntegerOverflow=on  OutDataTypeStr=Inherit: Same as input  ParamDataTypeStr=Inherit: Same as input
  Demux2 : Demux  Outputs=3
  In Case of singularity : Subsystem
  In Case of singularity1 : Subsystem
  Integrator1 : Integrator  InitialCondition=[p20(1), p20(2), p20(3)/180*pi]'
  Integrator2 : Integrator
  Mux3 : Mux  Inputs=3
  Rotation matrix in yaw : Subsystem
  Sum1 : Sum  Inputs=|++  InputSameDT=on  SaturateOnIntegerOverflow=on  OutDataTypeStr=Inherit: Same as first input
  Sum3 : Sum  Inputs=+-  InputSameDT=on  SaturateOnIntegerOverflow=on  OutDataTypeStr=Inherit: Same as first input
  "[-inf inf] to [-pi pi]1" : Subsystem
  inv(M1) : Gain  Gain=inv(M1+Ma1)  Multiplication=Matrix(K*u)  SaturateOnIntegerOverflow=on  OutDataTypeStr=Inherit: Same as input  ParamDataTypeStr=Inherit: Same as input
  p : Outport
  v : Outport  Port=2
  wires:
  Sum3/1 -> inv(M1)/1
  inv(M1)/1 -> In Case of singularity/1(input)
  Rotation matrix in yaw/1(R*nu) -> Integrator1/1
  " "/1 -> Rotation matrix in yaw/1(psi)
  tau/1 -> Sum3/1
  Integrator2/1 -> In Case of singularity1/1(input)
  In Case of singularity/1(output) -> Integrator2/1
  In Case of singularity1/1(output) -> Rotation matrix in yaw/2(nu), D/1, Coriolis and centripetal forces/1(nu), v/1
  D/1 -> Sum1/2
  Coriolis and centripetal forces/1(Output) -> Sum1/1
  Sum1/1 -> Sum3/2
  Demux2/3 -> "[-inf inf] to [-pi pi]1"/1(x [-inf inf])
  Integrator1/1 -> " "/1, Demux2/1
  "[-inf inf] to [-pi pi]1"/1(y [-pi pi]) -> Mux3/3
  Demux2/2 -> Mux3/2
  Demux2/1 -> Mux3/1
  Mux3/1 -> p/1

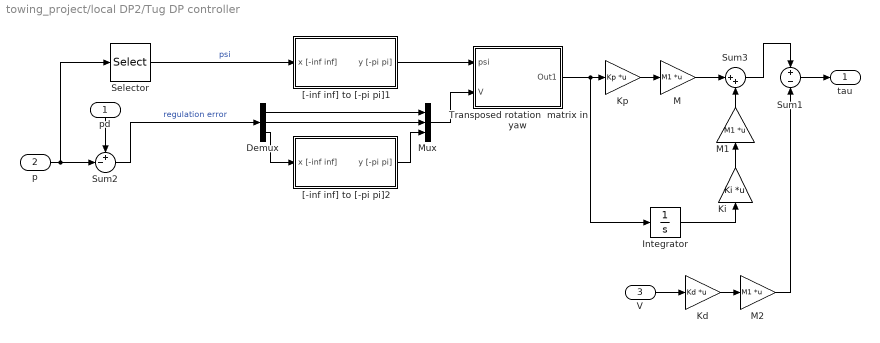
== system towing_project/local DP2/Tug DP controller ==
  pd : Inport
  p : Inport  Port=2
  V : Inport  Port=3
  Demux : Demux  Outputs=3
  Integrator : Integrator
  Kd : Gain  Gain=Kd  Multiplication=Matrix(K*u)  SaturateOnIntegerOverflow=on  OutDataTypeStr=Inherit: Same as input  ParamDataTypeStr=Inherit: Same as input
  Ki : Gain  Gain=Ki  Multiplication=Matrix(K*u)  SaturateOnIntegerOverflow=on  OutDataTypeStr=Inherit: Same as input  ParamDataTypeStr=Inherit: Same as input
  Kp : Gain  Gain=Kp  Multiplication=Matrix(K*u)  SaturateOnIntegerOverflow=on  OutDataTypeStr=Inherit: Same as input  ParamDataTypeStr=Inherit: Same as input
  M : Gain  Gain=M1  Multiplication=Matrix(K*u)  SaturateOnIntegerOverflow=on  OutDataTypeStr=Inherit: Same as input  ParamDataTypeStr=Inherit: Same as input
  M1 : Gain  Gain=M1  Multiplication=Matrix(K*u)  SaturateOnIntegerOverflow=on  OutDataTypeStr=Inherit: Same as input  ParamDataTypeStr=Inherit: Same as input
  M2 : Gain  Gain=M1  Multiplication=Matrix(K*u)  SaturateOnIntegerOverflow=on  OutDataTypeStr=Inherit: Same as input  ParamDataTypeStr=Inherit: Same as input
  Mux : Mux  Inputs=3
  Selector : Selector  InputPortWidth=3  IndexOptions=Index vector (dialog)  Indices=[ 3]  OutputSizes=1
  Sum1 : Sum  Inputs=+-  InputSameDT=on  SaturateOnIntegerOverflow=on  OutDataTypeStr=Inherit: Same as first input
  Sum2 : Sum  Inputs=+-|  InputSameDT=on  SaturateOnIntegerOverflow=on  OutDataTypeStr=Inherit: Same as first input
  Sum3 : Sum  Inputs=|++  InputSameDT=on  SaturateOnIntegerOverflow=on  OutDataTypeStr=Inherit: Same as first input
  Transposed rotation  matrix in yaw : Subsystem
  "[-inf inf] to [-pi pi]1" : Subsystem
  "[-inf inf] to [-pi pi]2" : Subsystem
  tau : Outport  InitialOutput=0
  wires:
  "[-inf inf] to [-pi pi]1"/1(y [-pi pi]) -> Transposed rotation  matrix in yaw/1(psi)
  Selector/1 -> "[-inf inf] to [-pi pi]1"/1(x [-inf inf])  "psi"
  Mux/1 -> Transposed rotation  matrix in yaw/2(V)
  Demux/1 -> Mux/1
  Demux/2 -> Mux/2
  "[-inf inf] to [-pi pi]2"/1(y [-pi pi]) -> Mux/3
  Sum2/1 -> Demux/1  "regulation error"
  Demux/3 -> "[-inf inf] to [-pi pi]2"/1(x [-inf inf])
  pd/1 -> Sum2/1
  Sum1/1 -> tau/1
  p/1 -> Sum2/2, Selector/1
  V/1 -> Kd/1
  Integrator/1 -> Ki/1
  Kp/1 -> M/1
  Ki/1 -> M1/1
  Transposed rotation  matrix in yaw/1(Out1) -> Kp/1, Integrator/1
  Kd/1 -> M2/1
  M/1 -> Sum3/1
  M1/1 -> Sum3/2
  Sum3/1 -> Sum1/1
  M2/1 -> Sum1/2

== system towing_project/local DP3/Propulsion system ==
  tau : Inport
  AzimuthAngle1 : ToWorkspace  VariableName=AziAng3  SampleTime=-1
  Gain : Gain  Gain=1/1000
  Gain1 : Gain  Gain=1000
  Level-2 MATLAB S-Function : M-S-Function  FunctionName=msfunTA_PA  Parameters=f0,a0,wa
  RealTau : ToWorkspace  VariableName=RealTau3  SampleTime=-1
  Terminator : Terminator
  Terminator1 : Terminator
  Terminator2 : Terminator
  ThrusterForce : ToWorkspace  VariableName=Thrust3  SampleTime=-1
  real tau : Outport
  thrusts : Outport  Port=2
  azimuth angles : Outport  Port=3
  wires:
  tau/1 -> Gain/1
  Level-2 MATLAB S-Function/2 -> Terminator/1
  Level-2 MATLAB S-Function/3 -> AzimuthAngle1/1, azimuth angles/1
  Level-2 MATLAB S-Function/4 -> Terminator1/1
  Level-2 MATLAB S-Function/5 -> Gain1/1
  Level-2 MATLAB S-Function/6 -> Terminator2/1
  Level-2 MATLAB S-Function/1 -> ThrusterForce/1, thrusts/1
  Gain/1 -> Level-2 MATLAB S-Function/1
  Gain1/1 -> RealTau/1, real tau/1

== system towing_project/local DP3/Tug ==
  note: nu_dot
  note: etadot
  tau : Inport
  " " : Selector  InputPortWidth=3  IndexOptions=Index vector (dialog)  Indices=[3]  OutputSizes=1
  Coriolis and centripetal forces : Subsystem
  D : Gain  Gain=D1  Multiplication=Matrix(K*u)  SaturateOnIntegerOverflow=on  OutDataTypeStr=Inherit: Same as input  ParamDataTypeStr=Inherit: Same as input
  Demux2 : Demux  Outputs=3
  In Case of singularity : Subsystem
  In Case of singularity1 : Subsystem
  Integrator1 : Integrator  InitialCondition=[p30(1), p30(2), p30(3)/180*pi]'
  Integrator2 : Integrator
  Mux3 : Mux  Inputs=3
  Rotation matrix in yaw : Subsystem
  Sum1 : Sum  Inputs=|++  InputSameDT=on  SaturateOnIntegerOverflow=on  OutDataTypeStr=Inherit: Same as first input
  Sum3 : Sum  Inputs=+-  InputSameDT=on  SaturateOnIntegerOverflow=on  OutDataTypeStr=Inherit: Same as first input
  "[-inf inf] to [-pi pi]1" : Subsystem
  inv(M1) : Gain  Gain=inv(M1+Ma1)  Multiplication=Matrix(K*u)  SaturateOnIntegerOverflow=on  OutDataTypeStr=Inherit: Same as input  ParamDataTypeStr=Inherit: Same as input
  p : Outport
  v : Outport  Port=2
  wires:
  Sum3/1 -> inv(M1)/1
  inv(M1)/1 -> In Case of singularity/1(input)
  Rotation matrix in yaw/1(R*nu) -> Integrator1/1
  Integrator1/1 -> Demux2/1, " "/1
  " "/1 -> Rotation matrix in yaw/1(psi)
  tau/1 -> Sum3/1
  Integrator2/1 -> In Case of singularity1/1(input)
  In Case of singularity/1(output) -> Integrator2/1
  In Case of singularity1/1(output) -> Rotation matrix in yaw/2(nu), D/1, Coriolis and centripetal forces/1(nu), v/1
  D/1 -> Sum1/2
  Coriolis and centripetal forces/1(Output) -> Sum1/1
  Sum1/1 -> Sum3/2
  Demux2/3 -> "[-inf inf] to [-pi pi]1"/1(x [-inf inf])
  Demux2/1 -> Mux3/1
  Demux2/2 -> Mux3/2
  "[-inf inf] to [-pi pi]1"/1(y [-pi pi]) -> Mux3/3
  Mux3/1 -> p/1

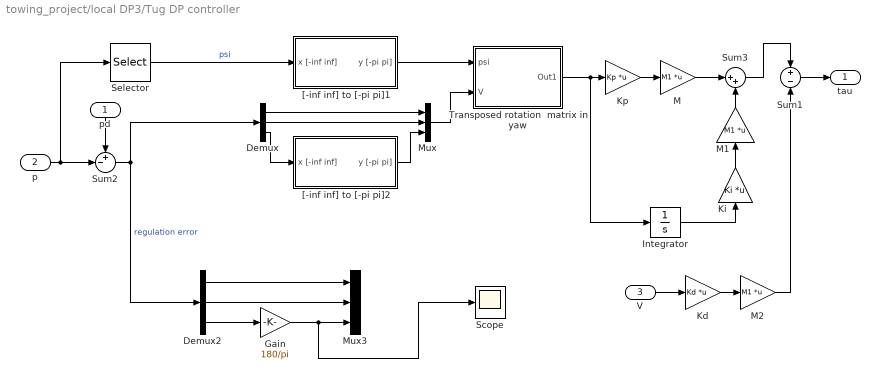
== system towing_project/local DP3/Tug DP controller ==
  pd : Inport
  p : Inport  Port=2
  V : Inport  Port=3
  Demux : Demux  Outputs=3
  Demux2 : Demux  Outputs=3
  Gain : Gain  Gain=180/pi
  Integrator : Integrator
  Kd : Gain  Gain=Kd  Multiplication=Matrix(K*u)  SaturateOnIntegerOverflow=on  OutDataTypeStr=Inherit: Same as input  ParamDataTypeStr=Inherit: Same as input
  Ki : Gain  Gain=Ki  Multiplication=Matrix(K*u)  SaturateOnIntegerOverflow=on  OutDataTypeStr=Inherit: Same as input  ParamDataTypeStr=Inherit: Same as input
  Kp : Gain  Gain=Kp  Multiplication=Matrix(K*u)  SaturateOnIntegerOverflow=on  OutDataTypeStr=Inherit: Same as input  ParamDataTypeStr=Inherit: Same as input
  M : Gain  Gain=M1  Multiplication=Matrix(K*u)  SaturateOnIntegerOverflow=on  OutDataTypeStr=Inherit: Same as input  ParamDataTypeStr=Inherit: Same as input
  M1 : Gain  Gain=M1  Multiplication=Matrix(K*u)  SaturateOnIntegerOverflow=on  OutDataTypeStr=Inherit: Same as input  ParamDataTypeStr=Inherit: Same as input
  M2 : Gain  Gain=M1  Multiplication=Matrix(K*u)  SaturateOnIntegerOverflow=on  OutDataTypeStr=Inherit: Same as input  ParamDataTypeStr=Inherit: Same as input
  Mux : Mux  Inputs=3
  Mux3 : Mux  Inputs=3
  Scope : Scope
  Selector : Selector  InputPortWidth=3  IndexOptions=Index vector (dialog)  Indices=[ 3]  OutputSizes=1
  Sum1 : Sum  Inputs=+-  InputSameDT=on  SaturateOnIntegerOverflow=on  OutDataTypeStr=Inherit: Same as first input
  Sum2 : Sum  Inputs=+-|  InputSameDT=on  SaturateOnIntegerOverflow=on  OutDataTypeStr=Inherit: Same as first input
  Sum3 : Sum  Inputs=|++  InputSameDT=on  SaturateOnIntegerOverflow=on  OutDataTypeStr=Inherit: Same as first input
  Transposed rotation  matrix in yaw : Subsystem
  "[-inf inf] to [-pi pi]1" : Subsystem
  "[-inf inf] to [-pi pi]2" : Subsystem
  tau : Outport  InitialOutput=0
  wires:
  "[-inf inf] to [-pi pi]1"/1(y [-pi pi]) -> Transposed rotation  matrix in yaw/1(psi)
  Selector/1 -> "[-inf inf] to [-pi pi]1"/1(x [-inf inf])  "psi"
  Mux/1 -> Transposed rotation  matrix in yaw/2(V)
  Demux/1 -> Mux/1
  Demux/2 -> Mux/2
  "[-inf inf] to [-pi pi]2"/1(y [-pi pi]) -> Mux/3
  Sum2/1 -> Demux2/1, Demux/1  "regulation error"
  Demux/3 -> "[-inf inf] to [-pi pi]2"/1(x [-inf inf])
  pd/1 -> Sum2/1
  Sum1/1 -> tau/1
  p/1 -> Sum2/2, Selector/1
  V/1 -> Kd/1
  Integrator/1 -> Ki/1
  Kp/1 -> M/1
  Ki/1 -> M1/1
  Transposed rotation  matrix in yaw/1(Out1) -> Kp/1, Integrator/1
  Kd/1 -> M2/1
  M/1 -> Sum3/1
  M1/1 -> Sum3/2
  Sum3/1 -> Sum1/1
  M2/1 -> Sum1/2
  Demux2/3 -> Gain/1
  Demux2/1 -> Mux3/1
  Demux2/2 -> Mux3/2
  Gain/1 -> Scope/1, Mux3/3

== system towing_project/local DP4/Propulsion system ==
  tau : Inport
  AzimuthAngle1 : ToWorkspace  VariableName=AziAng4  SampleTime=-1
  Gain : Gain  Gain=1/1000
  Gain1 : Gain  Gain=1000
  Level-2 MATLAB S-Function : M-S-Function  FunctionName=msfunTA_PA  Parameters=f0,a0,wa
  RealTau : ToWorkspace  VariableName=RealTau4  SampleTime=-1
  Terminator : Terminator
  Terminator1 : Terminator
  Terminator2 : Terminator
  ThrusterForce : ToWorkspace  VariableName=Thrust4  SampleTime=-1
  real tau : Outport
  thrusts : Outport  Port=2
  azimuth angles : Outport  Port=3
  wires:
  tau/1 -> Gain/1
  Level-2 MATLAB S-Function/2 -> Terminator/1
  Level-2 MATLAB S-Function/3 -> AzimuthAngle1/1, azimuth angles/1
  Level-2 MATLAB S-Function/4 -> Terminator1/1
  Level-2 MATLAB S-Function/5 -> Gain1/1
  Level-2 MATLAB S-Function/6 -> Terminator2/1
  Level-2 MATLAB S-Function/1 -> ThrusterForce/1, thrusts/1
  Gain/1 -> Level-2 MATLAB S-Function/1
  Gain1/1 -> RealTau/1, real tau/1

== system towing_project/local DP4/Tug ==
  note: nu_dot
  note: etadot
  tau : Inport
  " " : Selector  InputPortWidth=3  IndexOptions=Index vector (dialog)  Indices=[3]  OutputSizes=1
  Coriolis and centripetal forces : Subsystem
  D : Gain  Gain=D1  Multiplication=Matrix(K*u)  SaturateOnIntegerOverflow=on  OutDataTypeStr=Inherit: Same as input  ParamDataTypeStr=Inherit: Same as input
  Demux2 : Demux  Outputs=3
  In Case of singularity : Subsystem
  In Case of singularity1 : Subsystem
  Integrator1 : Integrator  InitialCondition=[p40(1), p40(2), p40(3)/180*pi]'
  Integrator2 : Integrator
  Mux3 : Mux  Inputs=3
  Rotation matrix in yaw : Subsystem
  Sum1 : Sum  Inputs=|++  InputSameDT=on  SaturateOnIntegerOverflow=on  OutDataTypeStr=Inherit: Same as first input
  Sum3 : Sum  Inputs=+-  InputSameDT=on  SaturateOnIntegerOverflow=on  OutDataTypeStr=Inherit: Same as first input
  "[-inf inf] to [-pi pi]1" : Subsystem
  inv(M1) : Gain  Gain=inv(M1+Ma1)  Multiplication=Matrix(K*u)  SaturateOnIntegerOverflow=on  OutDataTypeStr=Inherit: Same as input  ParamDataTypeStr=Inherit: Same as input
  p : Outport
  v : Outport  Port=2
  wires:
  Sum3/1 -> inv(M1)/1
  inv(M1)/1 -> In Case of singularity/1(input)
  Rotation matrix in yaw/1(R*nu) -> Integrator1/1
  Integrator1/1 -> Demux2/1, " "/1
  " "/1 -> Rotation matrix in yaw/1(psi)
  tau/1 -> Sum3/1
  Integrator2/1 -> In Case of singularity1/1(input)
  In Case of singularity/1(output) -> Integrator2/1
  In Case of singularity1/1(output) -> Rotation matrix in yaw/2(nu), D/1, Coriolis and centripetal forces/1(nu), v/1
  D/1 -> Sum1/2
  Coriolis and centripetal forces/1(Output) -> Sum1/1
  Sum1/1 -> Sum3/2
  Demux2/3 -> "[-inf inf] to [-pi pi]1"/1(x [-inf inf])
  Demux2/1 -> Mux3/1
  Demux2/2 -> Mux3/2
  "[-inf inf] to [-pi pi]1"/1(y [-pi pi]) -> Mux3/3
  Mux3/1 -> p/1

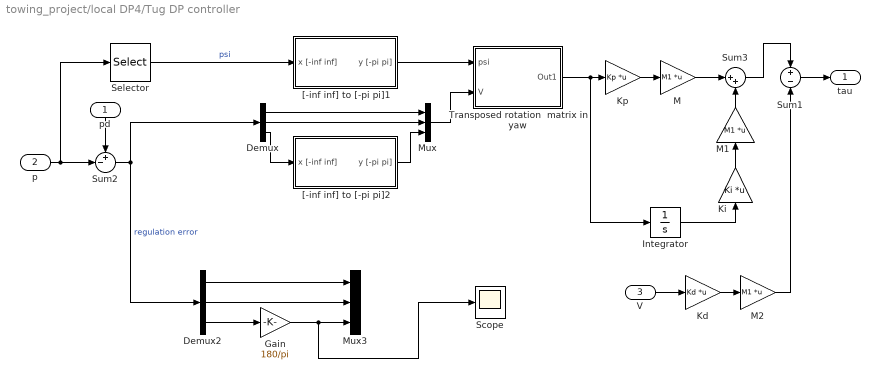
== system towing_project/local DP4/Tug DP controller ==
  pd : Inport
  p : Inport  Port=2
  V : Inport  Port=3
  Demux : Demux  Outputs=3
  Demux2 : Demux  Outputs=3
  Gain : Gain  Gain=180/pi
  Integrator : Integrator
  Kd : Gain  Gain=Kd  Multiplication=Matrix(K*u)  SaturateOnIntegerOverflow=on  OutDataTypeStr=Inherit: Same as input  ParamDataTypeStr=Inherit: Same as input
  Ki : Gain  Gain=Ki  Multiplication=Matrix(K*u)  SaturateOnIntegerOverflow=on  OutDataTypeStr=Inherit: Same as input  ParamDataTypeStr=Inherit: Same as input
  Kp : Gain  Gain=Kp  Multiplication=Matrix(K*u)  SaturateOnIntegerOverflow=on  OutDataTypeStr=Inherit: Same as input  ParamDataTypeStr=Inherit: Same as input
  M : Gain  Gain=M1  Multiplication=Matrix(K*u)  SaturateOnIntegerOverflow=on  OutDataTypeStr=Inherit: Same as input  ParamDataTypeStr=Inherit: Same as input
  M1 : Gain  Gain=M1  Multiplication=Matrix(K*u)  SaturateOnIntegerOverflow=on  OutDataTypeStr=Inherit: Same as input  ParamDataTypeStr=Inherit: Same as input
  M2 : Gain  Gain=M1  Multiplication=Matrix(K*u)  SaturateOnIntegerOverflow=on  OutDataTypeStr=Inherit: Same as input  ParamDataTypeStr=Inherit: Same as input
  Mux : Mux  Inputs=3
  Mux3 : Mux  Inputs=3
  Scope : Scope
  Selector : Selector  InputPortWidth=3  IndexOptions=Index vector (dialog)  Indices=[ 3]  OutputSizes=1
  Sum1 : Sum  Inputs=+-  InputSameDT=on  SaturateOnIntegerOverflow=on  OutDataTypeStr=Inherit: Same as first input
  Sum2 : Sum  Inputs=+-|  InputSameDT=on  SaturateOnIntegerOverflow=on  OutDataTypeStr=Inherit: Same as first input
  Sum3 : Sum  Inputs=|++  InputSameDT=on  SaturateOnIntegerOverflow=on  OutDataTypeStr=Inherit: Same as first input
  Transposed rotation  matrix in yaw : Subsystem
  "[-inf inf] to [-pi pi]1" : Subsystem
  "[-inf inf] to [-pi pi]2" : Subsystem
  tau : Outport  InitialOutput=0
  wires:
  "[-inf inf] to [-pi pi]1"/1(y [-pi pi]) -> Transposed rotation  matrix in yaw/1(psi)
  Selector/1 -> "[-inf inf] to [-pi pi]1"/1(x [-inf inf])  "psi"
  Mux/1 -> Transposed rotation  matrix in yaw/2(V)
  Demux/1 -> Mux/1
  Demux/2 -> Mux/2
  "[-inf inf] to [-pi pi]2"/1(y [-pi pi]) -> Mux/3
  Sum2/1 -> Demux2/1, Demux/1  "regulation error"
  Demux/3 -> "[-inf inf] to [-pi pi]2"/1(x [-inf inf])
  pd/1 -> Sum2/1
  Sum1/1 -> tau/1
  p/1 -> Sum2/2, Selector/1
  V/1 -> Kd/1
  Integrator/1 -> Ki/1
  Kp/1 -> M/1
  Ki/1 -> M1/1
  Transposed rotation  matrix in yaw/1(Out1) -> Kp/1, Integrator/1
  Kd/1 -> M2/1
  M/1 -> Sum3/1
  M1/1 -> Sum3/2
  Sum3/1 -> Sum1/1
  M2/1 -> Sum1/2
  Demux2/3 -> Gain/1
  Demux2/1 -> Mux3/1
  Demux2/2 -> Mux3/2
  Gain/1 -> Scope/1, Mux3/3

== system towing_project/virtual leader---PID/Transposed rotation  matrix in yaw ==
  psi : Inport
  V : Inport  Port=2
  Mux : Mux  Inputs=2
  Mux1 : Mux  Inputs=3
  Row1 : Fcn  Expr=cos(u(1))*u(2)-sin(u(1))*u(3)
  Row2 : Fcn  Expr=sin(u(1))*u(2)+cos(u(1))*u(3)
  Row3 : Fcn  Expr=u(4)
  Out1 : Outport
  wires:
  Mux/1 -> Row3/1, Row2/1, Row1/1
  Row1/1 -> Mux1/1
  Row2/1 -> Mux1/2
  Row3/1 -> Mux1/3
  Mux1/1 -> Out1/1
  psi/1 -> Mux/1
  V/1 -> Mux/2

== system towing_project/virtual leader---PID/[-inf inf] to [-pi pi]1 ==
  note: x
  note: r
  x [-inf inf] : Inport
  Constant : Constant  Value=2*pi
  Gain : Gain  Gain=pi  SaturateOnIntegerOverflow=on  OutDataTypeStr=Inherit: Same as input  ParamDataTypeStr=Inherit: Same as input
  Math Function : Math  Operator=rem  SignedPower=on  SaturateOnIntegerOverflow=on
  Saturation : Saturate  UpperLimit=1e10  LowerLimit=-1e10
  Sign : Signum
  Sum : Sum  Inputs=|+-  SaturateOnIntegerOverflow=on
  Sum1 : Sum  Inputs=|++  SaturateOnIntegerOverflow=on
  y [-pi pi] : Outport
  wires:
  x [-inf inf]/1 -> Saturation/1
  Sign/1 -> Gain/1
  Gain/1 -> Sum/2, Sum1/2
  Sum1/1 -> Math Function/1
  Constant/1 -> Math Function/2
  Math Function/1 -> Sum/1
  Sum/1 -> y [-pi pi]/1
  Saturation/1 -> Sum1/1, Sign/1

== system towing_project/virtual leader---PID/[-inf inf] to [-pi pi]2 ==
  note: r
  note: x
  x [-inf inf] : Inport
  Constant : Constant  Value=2*pi
  Gain : Gain  Gain=pi  SaturateOnIntegerOverflow=on  OutDataTypeStr=Inherit: Same as input  ParamDataTypeStr=Inherit: Same as input
  Math Function : Math  Operator=rem  SignedPower=on  SaturateOnIntegerOverflow=on
  Saturation : Saturate  UpperLimit=1e10  LowerLimit=-1e10
  Sign : Signum
  Sum : Sum  Inputs=|+-  SaturateOnIntegerOverflow=on
  Sum1 : Sum  Inputs=|++  SaturateOnIntegerOverflow=on
  y [-pi pi] : Outport
  wires:
  Saturation/1 -> Sign/1, Sum1/1
  Sum/1 -> y [-pi pi]/1
  Math Function/1 -> Sum/1
  Constant/1 -> Math Function/2
  Sum1/1 -> Math Function/1
  Gain/1 -> Sum1/2, Sum/2
  Sign/1 -> Gain/1
  x [-inf inf]/1 -> Saturation/1

== system towing_project/MotherShip/Coriolis and centripetal forces/Subsystem ==
  v : Inport
  r : Inport  Port=2
  -a22 : Gain  Gain=-M(2,2)-Ma(2,2)  Multiplication=Matrix(K*u)  SaturateOnIntegerOverflow=on  OutDataTypeStr=Inherit: Same as input  ParamDataTypeStr=Inherit: Same as input
  -a26 : Gain  Gain=-M(2,3)-Ma(2,3)  Multiplication=Matrix(K*u)  SaturateOnIntegerOverflow=on  OutDataTypeStr=Inherit: Same as input  ParamDataTypeStr=Inherit: Same as input
  Add : Sum
  Math Function : Math  Operator=magnitude^2  SignedPower=on  SaturateOnIntegerOverflow=on
  Product : Product  RndMeth=Zero
  x direction : Outport
  wires:
  v/1 -> Product/1
  r/1 -> Product/2, Math Function/1
  Product/1 -> -a22/1
  Math Function/1 -> -a26/1
  -a22/1 -> Add/1
  -a26/1 -> Add/2
  Add/1 -> x direction/1

== system towing_project/MotherShip/Coriolis and centripetal forces/Subsystem1 ==
  u : Inport
  r : Inport  Port=2
  Product : Product  RndMeth=Zero
  a11 : Gain  Gain=M(1,1)+Ma(1,1)  Multiplication=Matrix(K*u)  SaturateOnIntegerOverflow=on  OutDataTypeStr=Inherit: Same as input  ParamDataTypeStr=Inherit: Same as input
  y direction : Outport
  wires:
  Product/1 -> a11/1
  r/1 -> Product/2
  u/1 -> Product/1
  a11/1 -> y direction/1

== system towing_project/MotherShip/Coriolis and centripetal forces/Subsystem2 ==
  u : Inport
  v : Inport  Port=2
  r : Inport  Port=3
  Add : Sum
  Add1 : Sum  Inputs=+-
  Product : Product  RndMeth=Zero
  Product1 : Product  RndMeth=Zero
  a11 : Gain  Gain=M(1,1)+Ma(1,1)  Multiplication=Matrix(K*u)  SaturateOnIntegerOverflow=on  OutDataTypeStr=Inherit: Same as input  ParamDataTypeStr=Inherit: Same as input
  a22 : Gain  Gain=M(2,2)+Ma(2,2)  Multiplication=Matrix(K*u)  SaturateOnIntegerOverflow=on  OutDataTypeStr=Inherit: Same as input  ParamDataTypeStr=Inherit: Same as input
  a62 : Gain  Gain=M(3,2)+Ma(3,2)  Multiplication=Matrix(K*u)  SaturateOnIntegerOverflow=on  OutDataTypeStr=Inherit: Same as input  ParamDataTypeStr=Inherit: Same as input
  yaw direction : Outport
  wires:
  u/1 -> Product/1, Product1/1
  r/1 -> Product/2
  Product/1 -> a62/1
  v/1 -> Product1/2
  Product1/1 -> a22/1, a11/1
  a22/1 -> Add1/1
  a11/1 -> Add1/2
  Add1/1 -> Add/2
  a62/1 -> Add/1
  Add/1 -> yaw direction/1

== system towing_project/local DP1/Tug/Coriolis and centripetal forces ==
  nu : Inport
  Mux : Mux  Inputs=3
  Selector1 : Selector  InputPortWidth=3  IndexOptions=Index vector (dialog)  Indices=[1 ]  OutputSizes=1
  Selector2 : Selector  InputPortWidth=3  IndexOptions=Index vector (dialog)  Indices=[2]  OutputSizes=1
  Selector3 : Selector  InputPortWidth=3  IndexOptions=Index vector (dialog)  Indices=[3]  OutputSizes=1
  Subsystem : Subsystem
  Subsystem1 : Subsystem
  Subsystem2 : Subsystem
  Output : Outport
  wires:
  nu/1 -> Selector1/1, Selector2/1, Selector3/1
  Selector2/1 -> Subsystem/1(v), Subsystem2/2(v)  "v"
  Selector3/1 -> Subsystem/2(r), Subsystem1/2(r), Subsystem2/3(r)  "r"
  Selector1/1 -> Subsystem1/1(u), Subsystem2/1(u)  "u"
  Subsystem/1(x direction) -> Mux/1
  Subsystem1/1(y direction) -> Mux/2
  Subsystem2/1(yaw direction) -> Mux/3
  Mux/1 -> Output/1

== system towing_project/local DP1/Tug/In Case of singularity ==
  input : Inport
  Compare To Constant : simulink/Logic and Bit Operations/Compare To Constant  relop=>=  const=1e8  OutDataTypeStr=boolean
  Stop Simulation : Stop
  output : Outport
  wires:
  input/1 -> output/1, Compare To Constant/1
  Compare To Constant/1 -> Stop Simulation/1

== system towing_project/local DP1/Tug/In Case of singularity1 ==
  input : Inport
  Compare To Constant : simulink/Logic and Bit Operations/Compare To Constant  relop=>=  const=1e10  OutDataTypeStr=boolean
  Stop Simulation : Stop
  output : Outport
  wires:
  input/1 -> output/1, Compare To Constant/1
  Compare To Constant/1 -> Stop Simulation/1

== system towing_project/local DP1/Tug/Rotation matrix in yaw ==
  psi : Inport
  nu : Inport  Port=2
  Fcn : Fcn  Expr=cos(u(1))*u(2)-sin(u(1))*u(3)
  Fcn1 : Fcn  Expr=sin(u(1))*u(2)+cos(u(1))*u(3)
  Fcn2 : Fcn  Expr=u(4)
  Mux : Mux  Inputs=2
  Mux1 : Mux  Inputs=3
  R*nu : Outport
  wires:
  Mux1/1 -> R*nu/1  "eta_dot"
  Mux/1 -> Fcn/1, Fcn1/1, Fcn2/1
  psi/1 -> Mux/1
  nu/1 -> Mux/2
  Fcn1/1 -> Mux1/2  "y_dot"
  Fcn/1 -> Mux1/1  "x_dot"
  Fcn2/1 -> Mux1/3  "psi_dot"

== system towing_project/local DP1/Tug/[-inf inf] to [-pi pi]1 ==
  note: x
  note: r
  x [-inf inf] : Inport
  Constant : Constant  Value=2*pi
  Gain : Gain  Gain=pi  SaturateOnIntegerOverflow=on  OutDataTypeStr=Inherit: Same as input  ParamDataTypeStr=Inherit: Same as input
  Math Function : Math  Operator=rem  SignedPower=on  SaturateOnIntegerOverflow=on
  Saturation : Saturate  UpperLimit=1e10  LowerLimit=-1e10
  Sign : Signum
  Sum : Sum  Inputs=|+-  SaturateOnIntegerOverflow=on
  Sum1 : Sum  Inputs=|++  SaturateOnIntegerOverflow=on
  y [-pi pi] : Outport
  wires:
  x [-inf inf]/1 -> Saturation/1
  Sign/1 -> Gain/1
  Gain/1 -> Sum/2, Sum1/2
  Sum1/1 -> Math Function/1
  Constant/1 -> Math Function/2
  Math Function/1 -> Sum/1
  Sum/1 -> y [-pi pi]/1
  Saturation/1 -> Sum1/1, Sign/1
